simulink model "EngBrk_ECRCtl"  (R2016b)
settings: configuration reference "CodeGenConfigSet" (kept outside this file)
values from neighbouring files (symbols this model uses):
  EngBrk_pECRBstDflVal_C = Calibration.Parameter    [init_EngBrk_ECRCtl.m]
  EngBrk_pECRBstOff_C = Calibration.Parameter    [init_EngBrk_ECRCtl.m]
  EngBrk_pECRBstOn_C = Calibration.Parameter    [init_EngBrk_ECRCtl.m]
  EngBrk_tiECRBstOff_C = Calibration.Parameter    [init_EngBrk_ECRCtl.m]
  EngBrk_tiECRBstOn_C = Calibration.Parameter    [init_EngBrk_ECRCtl.m]
  PRC_100 = uint8(100)    [init_EngBrk_ECRCtl.m]
  PRC_ZERO = uint8(0)    [init_EngBrk_ECRCtl.m]
undefined symbols (not defined in the file or in its folder): EngBrk_ECRCtl_DT
settings Model: Creator=lenovo  LastModifiedBy=lenovo
settings ConfigSetRef: SourceLocation=Base Workspace

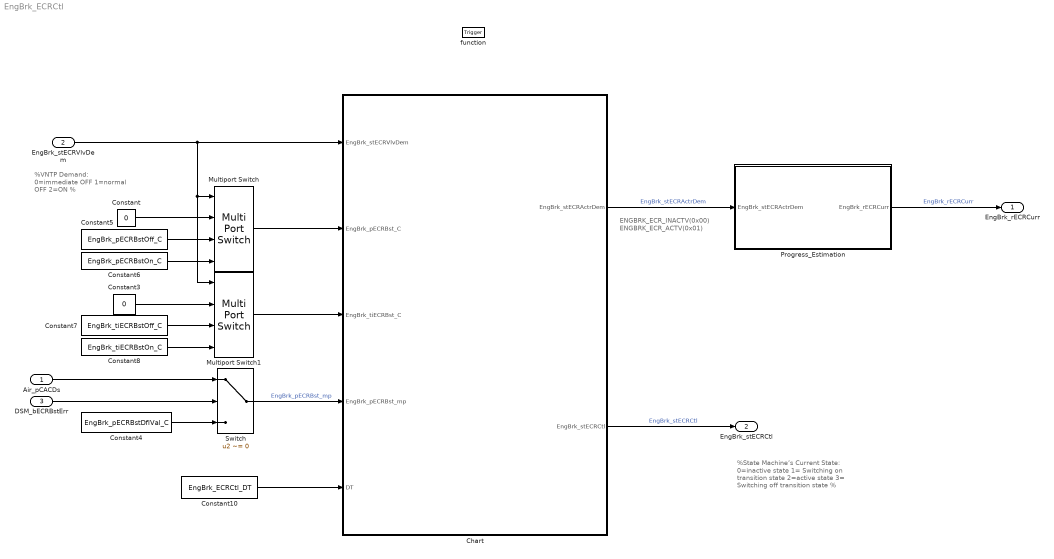
== system EngBrk_ECRCtl ==
  note: ENGBRK_ECR_INACTV(0x00)
      | ENGBRK_ECR_ACTV(0x01)
  note: %VNTP Demand:
      | 0=immediate OFF
      | 1=normal OFF
      | 2=ON %
  note: %State Machine’s Current State:
      | 0=inactive state
      | 1= Switching on transition state
      | 2=active state
      | 3= Switching off transition state %
  Air_pCACDs : Inport  Tag=kPa  Description=Air pressure downstream of the charge air cooler  OutMin=-3276.8  OutMax=3276.7  OutDataTypeStr=AirPressure_kPa
  EngBrk_stECRVlvDem : Inport  Description=Activation demand to Engine compression release Valve(ECRVlv)  Port=2  OutMin=0  OutMax=255  OutDataTypeStr=State_uint8
  DSM_bECRBstErr : Inport  Description=state of FId_ECRBstErr  Port=3  OutMin=0  OutMax=1  OutDataTypeStr=boolean
  function : TriggerPort  TriggerType=function-call  VariantControl=Variant
  Chart : Stateflow chart  TreatAsAtomicUnit=on
  Constant : Constant  Value=0  OutDataTypeStr=Inherit: Inherit via back propagation
  Constant10 : Constant  Value=EngBrk_ECRCtl_DT  OutDataTypeStr=Inherit: Inherit via back propagation
  Constant3 : Constant  Value=0  OutDataTypeStr=Inherit: Inherit via back propagation
  Constant4 : Constant  Value=EngBrk_pECRBstDflVal_C
  Constant5 : Constant  Value=EngBrk_pECRBstOff_C
  Constant6 : Constant  Value=EngBrk_pECRBstOn_C
  Constant7 : Constant  Value=EngBrk_tiECRBstOff_C
  Constant8 : Constant  Value=EngBrk_tiECRBstOn_C
  Multiport Switch : MultiPortSwitch  DataPortOrder=Zero-based contiguous  SaturateOnIntegerOverflow=on  InputSameDT=on
  Multiport Switch1 : MultiPortSwitch  DataPortOrder=Zero-based contiguous  SaturateOnIntegerOverflow=on  InputSameDT=on
  Progress_Estimation : Subsystem
  Switch : Switch  Criteria=u2 ~= 0  SaturateOnIntegerOverflow=on  InputSameDT=on
  EngBrk_rECRCurr : Outport  Tag=%  Description=Current status of the Engine compression release Valve(ECRVlv) state machine  OutMin=-200  OutMax=200  OutDataTypeStr=DutyCycle_rate
  EngBrk_stECRCtl : Outport  Description=Current status of the Engine compression release Valve(ECRVlv)  Port=2  OutMin=0  OutMax=255  OutDataTypeStr=State_uint8
  wires:
  Constant10/1 -> Chart/5(DT)
  Chart/1(EngBrk_stECRActrDem) -> Progress_Estimation/1(EngBrk_stECRActrDem)  "EngBrk_stECRActrDem"
  DSM_bECRBstErr/1 -> Switch/2
  Constant/1 -> Multiport Switch/2
  EngBrk_stECRVlvDem/1 -> Chart/1(EngBrk_stECRVlvDem), Multiport Switch/1, Multiport Switch1/1
  Constant6/1 -> Multiport Switch/4
  Progress_Estimation/1(EngBrk_rECRCurr) -> EngBrk_rECRCurr/1  "EngBrk_rECRCurr"
  Chart/2(EngBrk_stECRCtl) -> EngBrk_stECRCtl/1  "EngBrk_stECRCtl"
  Constant4/1 -> Switch/3
  Constant7/1 -> Multiport Switch1/3
  Constant5/1 -> Multiport Switch/3
  Air_pCACDs/1 -> Switch/1
  Constant8/1 -> Multiport Switch1/4
  Multiport Switch/1 -> Chart/2(EngBrk_pECRBst_C)
  Constant3/1 -> Multiport Switch1/2
  Multiport Switch1/1 -> Chart/3(EngBrk_tiECRBst_C)
  Switch/1 -> Chart/4(EngBrk_pECRBst_mp)  "EngBrk_pECRBst_mp"

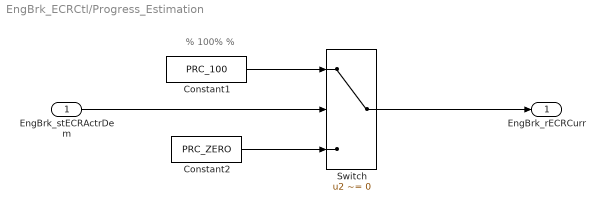
== system EngBrk_ECRCtl/Progress_Estimation ==
  note: % 100% %
  EngBrk_stECRActrDem : Inport
  Constant1 : Constant  Value=PRC_100  OutDataTypeStr=Inherit: Inherit via back propagation
  Constant2 : Constant  Value=PRC_ZERO  OutDataTypeStr=Inherit: Inherit via back propagation
  Switch : Switch  Criteria=u2 ~= 0  SaturateOnIntegerOverflow=on  InputSameDT=on
  EngBrk_rECRCurr : Outport
  wires:
  Constant1/1 -> Switch/1
  EngBrk_stECRActrDem/1 -> Switch/2
  Constant2/1 -> Switch/3
  Switch/1 -> EngBrk_rECRCurr/1

== stateflow chart EngBrk_ECRCtl/Chart ==
  state ENGBRK_ECR_WAIT_BSTOFF_OR_TO
    during:EngBrk_stECRCtl = 3;
    EngBrk_stECRActrDem = 1;
    timeout = timeout + DT;
  state ENGBRK_ECR_WAIT_ON_REQ
    during:EngBrk_stECRCtl = 0;
    EngBrk_stECRActrDem = 0;
    timeout = 0;
  state ENGBRK_ECR_WAIT_SHOFF_REQ
    during:EngBrk_stECRCtl = 2;
    EngBrk_stECRActrDem = 1;
    timeout = 0;
  state ENGBRK_ECR_WAIT_BSTON_OR_TO
    during:EngBrk_stECRCtl = 1;
    EngBrk_stECRActrDem = 0;
    timeout = timeout + DT;
  (default) -> ENGBRK_ECR_WAIT_ON_REQ
  ENGBRK_ECR_WAIT_BSTOFF_OR_TO -> ENGBRK_ECR_WAIT_ON_REQ [order 1] : [EngBrk_pECRBst_mp <= EngBrk_pECRBst_C...
      | || timeout >= EngBrk_tiECRBst_C...
      | || EngBrk_stECRVlvDem == 0]
  ENGBRK_ECR_WAIT_SHOFF_REQ -> ENGBRK_ECR_WAIT_ON_REQ [order 2] : [EngBrk_stECRVlvDem == 0]
  ENGBRK_ECR_WAIT_ON_REQ -> ENGBRK_ECR_WAIT_BSTON_OR_TO : [EngBrk_stECRVlvDem == 2]
  ENGBRK_ECR_WAIT_BSTON_OR_TO -> ENGBRK_ECR_WAIT_ON_REQ [order 1] : [EngBrk_stECRVlvDem != 2]
  ENGBRK_ECR_WAIT_BSTOFF_OR_TO -> ENGBRK_ECR_WAIT_SHOFF_REQ [order 2] : [EngBrk_stECRVlvDem == 2]
  ENGBRK_ECR_WAIT_SHOFF_REQ -> ENGBRK_ECR_WAIT_BSTOFF_OR_TO [order 1] : [EngBrk_stECRVlvDem == 1]
  ENGBRK_ECR_WAIT_BSTON_OR_TO -> ENGBRK_ECR_WAIT_SHOFF_REQ [order 2] : [EngBrk_pECRBst_mp <= EngBrk_pECRBst_C...
      | || timeout >= EngBrk_tiECRBst_C]
  data: EngBrk_stECRActrDem output; EngBrk_stECRCtl output; EngBrk_stECRVlvDem input; EngBrk_pECRBst_C input; EngBrk_tiECRBst_C input; EngBrk_pECRBst_mp input; timeout local uint16; DT input
